simulink model "SOGI_PLL_1ph"  (R2020a)
settings: Solver=ode3  StartTime=0.0  StopTime=1  FixedStep=0.000001  RelTol=1e-3
values from neighbouring files (symbols this model uses):
  A0 = 1    [SOGI_PLL_design.m]
  dA = 0.5    [SOGI_PLL_design.m]
  dphi = pi/4    (= 0.785398163397)    [SOGI_PLL_design.m]
  dw = 2*pi*2.5    (= 15.7079632679)    [SOGI_PLL_design.m]
  k = 9.2/w0/ts_SOGI    (= 1.46422547645)    [SOGI_PLL_design.m]
  Ki = Kp/Ti    [SOGI_PLL_design.m]
  Kp = 2/A0 * KP    [SOGI_PLL_design.m]
  tA = td + 0.75    (= 0.75)    [SOGI_PLL_design.m]
  tphi = td + 0.25    (= 0.25)    [SOGI_PLL_design.m]
  tw = td + 0.5    (= 0.5)    [SOGI_PLL_design.m]
  w0 = 2*pi*f0    (= 314.159265359)    [SOGI_PLL_design.m]
settings Model: Creator=Ulas  LastModifiedBy=ulask
settings SFSimCC: CustomCodeUndefinedFunction=UseInterfaceOnly

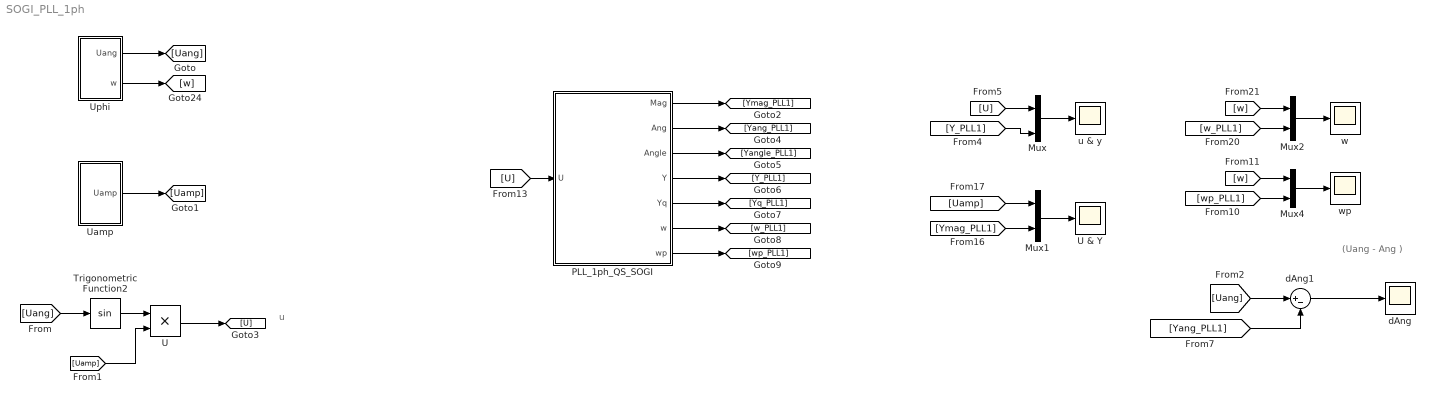
== system SOGI_PLL_1ph ==
  note: u
  note: (Uang - Ang )
  Mux{,1..2,4} (4 alike) : Mux  Inputs=2
  PLL_1ph_QS_SOGI : Subsystem
  Trigonometric Function2 : Trigonometry
  U : Product
  U & Y : Scope
  Uamp : Subsystem
  Uphi : Subsystem
  dAng : Scope
  dAng1 : Sum  Inputs=|+-
  u & y : Scope
  w : Scope
  wp : Scope
  wires:
  Mux/1 -> u & y/1
  [Uang] -> Trigonometric Function2/1
  Trigonometric Function2/1 -> U/1
  [Uamp] -> U/2
  [Uang] -> dAng1/1
  U/1 -> [U]
  [U] -> Mux/1
  Uphi/1(Uang) -> [Uang]
  Uamp/1(Uamp) -> [Uamp]
  [Yang_PLL1] -> dAng1/2
  [U] -> PLL_1ph_QS_SOGI/1(U)
  PLL_1ph_QS_SOGI/1(Mag) -> [Ymag_PLL1]
  PLL_1ph_QS_SOGI/4(Y) -> [Y_PLL1]
  PLL_1ph_QS_SOGI/3(Angle) -> [Yangle_PLL1]
  PLL_1ph_QS_SOGI/6(w) -> [w_PLL1]
  PLL_1ph_QS_SOGI/2(Ang) -> [Yang_PLL1]
  PLL_1ph_QS_SOGI/7(wp) -> [wp_PLL1]
  PLL_1ph_QS_SOGI/5(Yq) -> [Yq_PLL1]
  [Uamp] -> Mux1/1
  Mux1/1 -> U & Y/1
  [Ymag_PLL1] -> Mux1/2
  Uphi/2(w) -> [w]
  [w] -> Mux2/1
  Mux2/1 -> w/1
  [w_PLL1] -> Mux2/2
  dAng1/1 -> dAng/1
  [w] -> Mux4/1
  [wp_PLL1] -> Mux4/2
  Mux4/1 -> wp/1
  [Y_PLL1] -> Mux/2

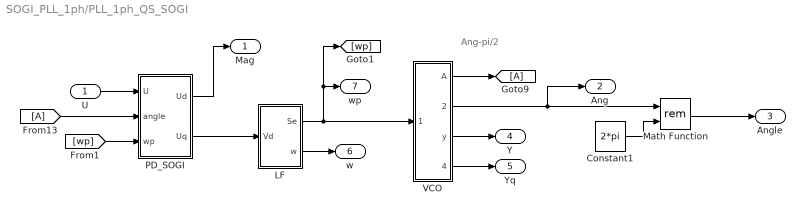
== system SOGI_PLL_1ph/PLL_1ph_QS_SOGI ==
  note: Ang-pi/2
  U : Inport
  Constant1 : Constant  Value=2*pi
  LF : Subsystem
  Math Function : Math  Operator=rem  SignedPower=on  SaturateOnIntegerOverflow=on
  PD_SOGI : Subsystem
  VCO : Subsystem
  Mag : Outport  VectorParamsAs1DForOutWhenUnconnected=off
  Ang : Outport  Port=2  VectorParamsAs1DForOutWhenUnconnected=off
  Angle : Outport  Port=3  VectorParamsAs1DForOutWhenUnconnected=off
  Y : Outport  Port=4  VectorParamsAs1DForOutWhenUnconnected=off
  Yq : Outport  Port=5  VectorParamsAs1DForOutWhenUnconnected=off
  w : Outport  Port=6  VectorParamsAs1DForOutWhenUnconnected=off
  wp : Outport  Port=7  VectorParamsAs1DForOutWhenUnconnected=off
  wires:
  VCO/2(ang) -> Ang/1, Math Function/1
  PD_SOGI/2(Uq) -> LF/1(Vd)
  VCO/3(y) -> Y/1
  LF/1(Se) -> [wp], wp/1, VCO/1(Se)
  [A] -> PD_SOGI/2(angle)
  Math Function/1 -> Angle/1
  VCO/1(A) -> [A]
  LF/2(w) -> w/1
  Constant1/1 -> Math Function/2
  U/1 -> PD_SOGI/1(U)
  VCO/4(yq) -> Yq/1
  PD_SOGI/1(Ud) -> Mag/1
  [wp] -> PD_SOGI/3(wp)

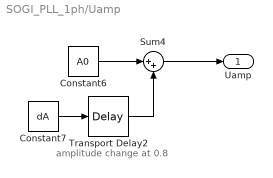
== system SOGI_PLL_1ph/Uamp ==
  note: amplitude change at 0.8
  Constant6 : Constant  Value=A0
  Constant7 : Constant  Value=dA
  Sum4 : Sum  Inputs=|++
  Transport Delay2 : TransportDelay  DelayTime=tA
  Uamp : Outport  VectorParamsAs1DForOutWhenUnconnected=off
  wires:
  Constant7/1 -> Transport Delay2/1
  Constant6/1 -> Sum4/1
  Sum4/1 -> Uamp/1
  Transport Delay2/1 -> Sum4/2

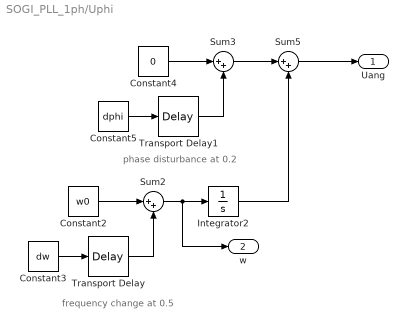
== system SOGI_PLL_1ph/Uphi ==
  note: frequency change at 0.5
  note: phase disturbance at 0.2
  Constant2 : Constant  Value=w0
  Constant3 : Constant  Value=dw
  Constant4 : Constant  Value=0
  Constant5 : Constant  Value=dphi
  Integrator2 : Integrator
  Sum2 : Sum  Inputs=|++
  Sum3 : Sum  Inputs=|++
  Sum5 : Sum  Inputs=|++
  Transport Delay : TransportDelay  DelayTime=tw
  Transport Delay1 : TransportDelay  DelayTime=tphi
  Uang : Outport  VectorParamsAs1DForOutWhenUnconnected=off
  w : Outport  Port=2  VectorParamsAs1DForOutWhenUnconnected=off
  wires:
  Integrator2/1 -> Sum5/2
  Constant5/1 -> Transport Delay1/1
  Sum2/1 -> w/1, Integrator2/1
  Sum5/1 -> Uang/1
  Constant3/1 -> Transport Delay/1
  Sum3/1 -> Sum5/1
  Transport Delay/1 -> Sum2/2
  Transport Delay1/1 -> Sum3/2
  Constant2/1 -> Sum2/1
  Constant4/1 -> Sum3/1

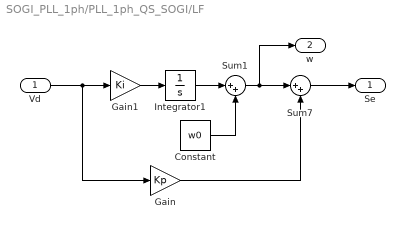
== system SOGI_PLL_1ph/PLL_1ph_QS_SOGI/LF ==
  Vd : Inport
  Constant : Constant  Value=w0
  Gain : Gain  Gain=Kp
  Gain1 : Gain  Gain=Ki
  Integrator1 : Integrator
  Sum1 : Sum  Inputs=|++
  Sum7 : Sum  Inputs=|++
  Se : Outport  VectorParamsAs1DForOutWhenUnconnected=off
  w : Outport  Port=2  VectorParamsAs1DForOutWhenUnconnected=off
  wires:
  Integrator1/1 -> Sum1/1
  Gain1/1 -> Integrator1/1
  Gain/1 -> Sum7/2
  Vd/1 -> Gain/1, Gain1/1
  Sum1/1 -> w/1, Sum7/1
  Constant/1 -> Sum1/2
  Sum7/1 -> Se/1

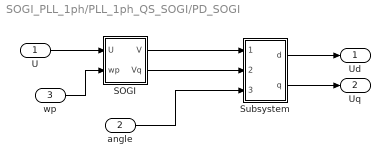
== system SOGI_PLL_1ph/PLL_1ph_QS_SOGI/PD_SOGI ==
  U : Inport
  angle : Inport  Port=2
  wp : Inport  Port=3
  SOGI : Subsystem
  Subsystem : Subsystem
  Ud : Outport  VectorParamsAs1DForOutWhenUnconnected=off
  Uq : Outport  Port=2  VectorParamsAs1DForOutWhenUnconnected=off
  wires:
  angle/1 -> Subsystem/3(angle)
  Subsystem/1(d) -> Ud/1
  Subsystem/2(q) -> Uq/1
  SOGI/2(Vq) -> Subsystem/2(beta)
  SOGI/1(V) -> Subsystem/1(alpha)
  U/1 -> SOGI/1(U)
  wp/1 -> SOGI/2(wp)

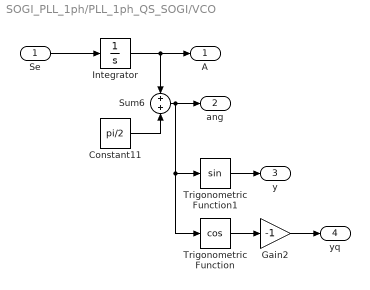
== system SOGI_PLL_1ph/PLL_1ph_QS_SOGI/VCO ==
  Se : Inport
  Constant11 : Constant  Value=pi/2
  Gain2 : Gain  Gain=-1
  Integrator : Integrator
  Sum6 : Sum
  Trigonometric Function : Trigonometry  Operator=cos
  Trigonometric Function1 : Trigonometry
  A : Outport  VectorParamsAs1DForOutWhenUnconnected=off
  ang : Outport  Port=2  VectorParamsAs1DForOutWhenUnconnected=off
  y : Outport  Port=3  VectorParamsAs1DForOutWhenUnconnected=off
  yq : Outport  Port=4  VectorParamsAs1DForOutWhenUnconnected=off
  wires:
  Se/1 -> Integrator/1
  Trigonometric Function/1 -> Gain2/1
  Integrator/1 -> Sum6/1, A/1
  Constant11/1 -> Sum6/2
  Trigonometric Function1/1 -> y/1
  Gain2/1 -> yq/1
  Sum6/1 -> Trigonometric Function/1, Trigonometric Function1/1, ang/1

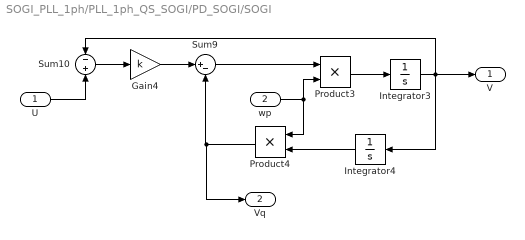
== system SOGI_PLL_1ph/PLL_1ph_QS_SOGI/PD_SOGI/SOGI ==
  U : Inport
  wp : Inport  Port=2
  Gain4 : Gain  Gain=k
  Integrator3 : Integrator
  Integrator4 : Integrator
  Product3 : Product
  Product4 : Product
  Sum10 : Sum  Inputs=-|+
  Sum9 : Sum  Inputs=|+-
  V : Outport  VectorParamsAs1DForOutWhenUnconnected=off
  Vq : Outport  Port=2  VectorParamsAs1DForOutWhenUnconnected=off
  wires:
  wp/1 -> Product3/2, Product4/1
  Integrator3/1 -> V/1, Sum10/1, Integrator4/1
  Sum9/1 -> Product3/1
  Sum10/1 -> Gain4/1
  Product3/1 -> Integrator3/1
  Gain4/1 -> Sum9/1
  Product4/1 -> Vq/1, Sum9/2
  Integrator4/1 -> Product4/2
  U/1 -> Sum10/2

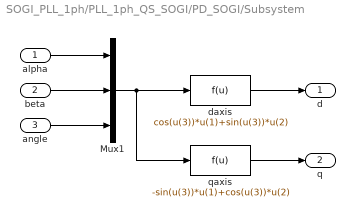
== system SOGI_PLL_1ph/PLL_1ph_QS_SOGI/PD_SOGI/Subsystem ==
  alpha : Inport
  beta : Inport  Port=2
  angle : Inport  Port=3
  Mux1 : Mux  Inputs=3
  daxis : Fcn  Expr=cos(u(3))*u(1)+sin(u(3))*u(2)
  qaxis : Fcn  Expr=-sin(u(3))*u(1)+cos(u(3))*u(2)
  d : Outport  VectorParamsAs1DForOutWhenUnconnected=off
  q : Outport  Port=2  VectorParamsAs1DForOutWhenUnconnected=off
  wires:
  Mux1/1 -> qaxis/1, daxis/1
  daxis/1 -> d/1
  angle/1 -> Mux1/3
  alpha/1 -> Mux1/1
  beta/1 -> Mux1/2
  qaxis/1 -> q/1
